simulink model "MODEL_FULL_SYSTEM"  (Simulink 7.8)
settings: Solver=ode1  StartTime=0.0  StopTime=inf  FixedStep=Ts  MaxStep=1e-3  RelTol=1e-3
PostLoadFcn:
  | Ts=80e-6; relays_settings_init;
InitFcn:
  | Ts=80e-6; relays_settings_init;
values from neighbouring files (symbols this model uses):
  relay_sets = xlsread('relay_settings_10272015.xlsx')    [relays_settings_init.m]
undefined symbols (not defined in the file or in its folder): dfilt, DiscIntNeverNeededParam, fdesignblkfcn, gcbh, Left, opmodbus_cb, ph, Right, type, V, X
libraries: simulink x72, modbus_lib x40, cables_lib x36, rtio_opalrt_common x21, rtlab x20, transformer_lib x13, dynamic_load_lib x12, powerlib x6, simulink_extras x6, ssn_lib x5, discretizing x4, rteventslib x4
(part 6 of 7)

== system MODEL_FULL_SYSTEM/SM_Master/Generator_09222015/Woodward Inputs/Speed_System ==
  In1 : Inport
  Clock1 : Clock
      settings: DisableCoverage=on
  Duty : Constant  DisableCoverage=on  Value=0.5
  Gain1 : Gain  Gain=5
  Gain3 : Gain  Gain=5
  Gain4 : Gain  Gain=1800
  Output : Trigonometry
  Product1 : Product  DisableCoverage=on  SaturateOnIntegerOverflow=on  InputSameDT=on  OutDataTypeStr=Inherit: Same as first input
  Product3 : Product  DisableCoverage=on  SaturateOnIntegerOverflow=on  InputSameDT=on  OutDataTypeStr=Inherit: Same as first input
  RTE Conversion : rteventslib/Signal Attributes/RTE Conversion  inputdatatype=RTE Boolean  outputdatatype=Double  compensation=Disabled  nbMaxEvents=10  sampleTime=Ts
  RTE SPWM : rteventslib/Sources/RTE SPWM  NumberPhases=1-ph  CenterAlignmentMode=On  MaxFreq=inf  MinFreq=0  EnablingPort=off  ComplementaryMode=off  SpaceVector=off  RiseTimeDelay=0  MaxEvents=10  SampleTime=Ts
  initialFreq : Constant  DisableCoverage=on  Value=2*pi
  Out1 : Outport
  wires:
  Gain1/1 -> Out1/1
  RTE Conversion/1 -> Gain1/1
  Duty/1 -> RTE SPWM/2
  RTE SPWM/1 -> RTE Conversion/1
  In1/1 -> Gain4/1
  Output/1 -> Gain3/1
  Gain4/1 -> RTE SPWM/1, Product3/2
  Product3/1 -> Product1/2
  initialFreq/1 -> Product3/1
  Clock1/1 -> Product1/1
  Product1/1 -> Output/1

== system MODEL_FULL_SYSTEM/SM_Master/Generator_09222015/Woodward Inputs/Speed_System1 ==
  In1 : Inport
  Clock1 : Clock
      settings: DisableCoverage=on
  Duty : Constant  DisableCoverage=on  Value=0.5
  Gain1 : Gain  Gain=5
  Gain3 : Gain  Gain=5
  Gain4 : Gain  Gain=1800
  Output : Trigonometry
  Product1 : Product  DisableCoverage=on  SaturateOnIntegerOverflow=on  InputSameDT=on  OutDataTypeStr=Inherit: Same as first input
  Product3 : Product  DisableCoverage=on  SaturateOnIntegerOverflow=on  InputSameDT=on  OutDataTypeStr=Inherit: Same as first input
  RTE Conversion : rteventslib/Signal Attributes/RTE Conversion  inputdatatype=RTE Boolean  outputdatatype=Double  compensation=Disabled  nbMaxEvents=10  sampleTime=Ts
  RTE SPWM : rteventslib/Sources/RTE SPWM  NumberPhases=1-ph  CenterAlignmentMode=On  MaxFreq=inf  MinFreq=0  EnablingPort=off  ComplementaryMode=off  SpaceVector=off  RiseTimeDelay=0  MaxEvents=10  SampleTime=Ts
  initialFreq : Constant  DisableCoverage=on  Value=2*pi
  Out1 : Outport
  wires:
  Gain1/1 -> Out1/1
  RTE Conversion/1 -> Gain1/1
  Duty/1 -> RTE SPWM/2
  RTE SPWM/1 -> RTE Conversion/1
  In1/1 -> Gain4/1
  Output/1 -> Gain3/1
  Gain4/1 -> RTE SPWM/1, Product3/2
  Product3/1 -> Product1/2
  initialFreq/1 -> Product3/1
  Clock1/1 -> Product1/1
  Product1/1 -> Output/1

== system MODEL_FULL_SYSTEM/SM_Master/Generator_09222015/Woodward Outputs/DIO - Gr3 ==
  Dout : Inport
  Bus Creator : BusCreator  Inputs=2
  Bus Selector : BusSelector  OutputSignals=DI_CH00-07  OutputAsBus=on
  Bus Selector1 : BusSelector  OutputSignals=DI_CH08-15  OutputAsBus=on
  Conditioning : Subsystem
  Conditioning1 : Subsystem
  DigitalIn : rtio_opalrt_common/DigitalIn  CtrlName='OpCtrl'  portNb=5  FcnNos=Slot 3 Module A Subsection 1  size=1  maxcount=8  count=8  sampleTime=0  numchan=8
      settings: AttributesFormatString=%<CtrlName>
  DigitalIn1 : rtio_opalrt_common/DigitalIn  CtrlName='OpCtrl'  portNb=6  FcnNos=Slot 3 Module A Subsection 2  size=1  maxcount=8  count=8  sampleTime=0  numchan=8
      settings: AttributesFormatString=%<CtrlName>
  DigitalOut : rtio_opalrt_common/DigitalOut  CtrlName='OpCtrl'  portNb=5  FcnNos=Slot 3 Module B Subsection 1  size=1  maxcount=8  count=8  numchan=8
      settings: AttributesFormatString=%<CtrlName>
  DigitalOut1 : rtio_opalrt_common/DigitalOut  CtrlName='OpCtrl'  portNb=6  FcnNos=Slot 3 Module B Subsection 2  size=1  maxcount=8  count=8  numchan=8
      settings: AttributesFormatString=%<CtrlName>
  Terminator{1,3,5..6} (4 alike) : Terminator
  DIn : Outport
  wires:
  DigitalOut/1 -> Terminator3/1
  DigitalOut1/1 -> Terminator1/1
  Dout/1 -> Bus Selector/1, Bus Selector1/1
  Bus Selector/1 -> DigitalOut/1
  Bus Selector1/1 -> DigitalOut1/1
  DigitalIn/2 -> Terminator5/1
  DigitalIn1/2 -> Terminator6/1
  DigitalIn/1 -> Conditioning/1(In1)  "DI_CH00-07"
  DigitalIn1/1 -> Conditioning1/1(In1)  "DI_CH08-15"
  Bus Creator/1 -> DIn/1
  Conditioning/1(Out1) -> Bus Creator/1
  Conditioning1/1(Out1) -> Bus Creator/2

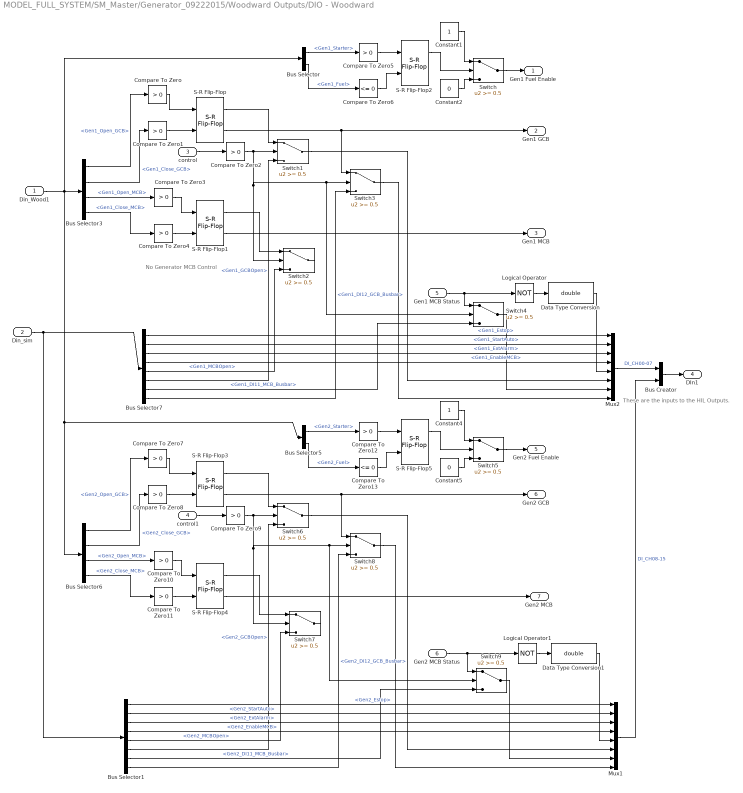
== system MODEL_FULL_SYSTEM/SM_Master/Generator_09222015/Woodward Outputs/DIO - Woodward ==
  note: No Generator MCB Control
  note: These are the inputs to
      | the HIL Outputs.
  Din_Wood1 : Inport
  Din_sim : Inport  Port=2
  control : Inport  Port=3
  control1 : Inport  Port=4
  Gen1 MCB Status : Inport  Port=5
  Gen2 MCB Status : Inport  Port=6
  Bus Creator : BusCreator  Inputs=2
  Bus Selector : BusSelector  OutputSignals=DI_CH00-07.Gen1_Starter,DI_CH00-07.Gen1_Fuel
  Bus Selector1 : BusSelector  OutputSignals=16 DOUT GR3.08-11.Gen2_Estop,16 DOUT GR3.08-11.Gen2_StartAuto,16 DOUT GR3.08-11.Gen2_ExtAlarm,16 DOUT GR3.08-11.Gen2_EnableMCB,16 DOUT GR3.12-15.Gen2_MCBOpen,16 DOUT GR3.12-15.Gen2_GCBOpen,16 DOUT GR3.12-15.Gen2_DI11_MCB_Busbar,16 DOUT GR3.12-15.Gen2_DI12_GCB_Busbar
  Bus Selector3 : BusSelector  OutputSignals=DI_CH00-07.Gen1_Open_GCB,DI_CH00-07.Gen1_Close_GCB,DI_CH00-07.Gen1_Open_MCB,DI_CH00-07.Gen1_Close_MCB
  Bus Selector5 : BusSelector  OutputSignals=DI_CH08-15.Gen2_Starter,DI_CH08-15.Gen2_Fuel
  Bus Selector6 : BusSelector  OutputSignals=DI_CH08-15.Gen2_Open_GCB,DI_CH08-15.Gen2_Close_GCB,DI_CH08-15.Gen2_Open_MCB,DI_CH08-15.Gen2_Close_MCB
  Bus Selector7 : BusSelector  OutputSignals=16 DOUT GR3.00-03.Gen1_Estop,16 DOUT GR3.00-03.Gen1_StartAuto,16 DOUT GR3.00-03.Gen1_ExtAlarm,16 DOUT GR3.00-03.Gen1_EnableMCB,16 DOUT GR3.04-07.Gen1_MCBOpen,16 DOUT GR3.04-07.Gen1_GCBOpen,16 DOUT GR3.04-07.Gen1_DI11_MCB_Busbar,16 DOUT GR3.04-07.Gen1_DI12_GCB_Busbar
  Compare To Zero{,1..5,7..12} (12 alike) : simulink/Logic and Bit Operations/Compare To Zero  relop=>  OutDataTypeStr=boolean
  Compare To Zero13 : simulink/Logic and Bit Operations/Compare To Zero  relop=<=  OutDataTypeStr=boolean
  Compare To Zero6 : simulink/Logic and Bit Operations/Compare To Zero  relop=<=  OutDataTypeStr=boolean
  Constant1 : Constant
  Constant2 : Constant  Value=0
  Constant4 : Constant
  Constant5 : Constant  Value=0
  Data Type Conversion : DataTypeConversion  OutDataTypeStr=double
  Data Type Conversion1 : DataTypeConversion  OutDataTypeStr=double
  Logical Operator : Logic  Operator=NOT  AllPortsSameDT=off  OutDataTypeStr=boolean
  Logical Operator1 : Logic  Operator=NOT  AllPortsSameDT=off  OutDataTypeStr=boolean
  Mux1 : Mux  Inputs=8
  Mux2 : Mux  Inputs=8
  S-R Flip-Flop{,1,3..4} (4 alike) : simulink_extras/Flip Flops/S-R Flip-Flop  initial_condition=1
  S-R Flip-Flop2 : simulink_extras/Flip Flops/S-R Flip-Flop  initial_condition=0
  S-R Flip-Flop5 : simulink_extras/Flip Flops/S-R Flip-Flop  initial_condition=0
  Switch : Switch  Threshold=0.5
  Switch{1..4,6..9} (8 alike) : Switch  Threshold=0.5  OutDataTypeStr=double
      Switch8 settings: LockScale=on
  Switch5 : Switch  Threshold=0.5
  Gen1 Fuel Enable : Outport
  Gen1 GCB : Outport  Port=2
  Gen1 MCB : Outport  Port=3
  DIn1 : Outport  Port=4
  Gen2 Fuel Enable : Outport  Port=5
  Gen2 GCB : Outport  Port=6
  Gen2 MCB : Outport  Port=7
  wires:
  S-R Flip-Flop1/2 -> Gen1 MCB/1
  Din_Wood1/1 -> Bus Selector3/1, Bus Selector/1, Bus Selector6/1, Bus Selector5/1
  control/1 -> Compare To Zero2/1
  Bus Creator/1 -> DIn1/1
  S-R Flip-Flop/1 -> Switch1/1
  Switch1/1 -> Mux2/6
  Bus Selector3/1 -> Compare To Zero/1  "<Gen1_Open_GCB>"
  Compare To Zero/1 -> S-R Flip-Flop/1
  Compare To Zero1/1 -> S-R Flip-Flop/2
  Bus Selector3/4 -> Compare To Zero4/1  "<Gen1_Close_MCB>"
  Compare To Zero4/1 -> S-R Flip-Flop1/2
  Compare To Zero3/1 -> S-R Flip-Flop1/1
  S-R Flip-Flop1/1 -> Switch2/1
  Compare To Zero2/1 -> Switch1/2, Switch2/2, Switch3/2, Switch4/2
  Mux1/1 -> Bus Creator/2  "DI_CH08-15"
  S-R Flip-Flop/2 -> Gen1 GCB/1, Switch3/1
  Bus Selector/1 -> Compare To Zero5/1  "<Gen1_Starter>"
  Bus Selector/2 -> Compare To Zero6/1  "<Gen1_Fuel>"
  S-R Flip-Flop2/1 -> Switch/2
  Compare To Zero5/1 -> S-R Flip-Flop2/1
  Constant2/1 -> Switch/3
  Constant1/1 -> Switch/1
  Compare To Zero6/1 -> S-R Flip-Flop2/2
  Switch/1 -> Gen1 Fuel Enable/1
  control1/1 -> Compare To Zero9/1
  S-R Flip-Flop3/1 -> Switch6/1
  Switch6/1 -> Mux1/6
  Bus Selector6/1 -> Compare To Zero7/1  "<Gen2_Open_GCB>"
  Compare To Zero7/1 -> S-R Flip-Flop3/1
  Compare To Zero8/1 -> S-R Flip-Flop3/2
  Bus Selector6/4 -> Compare To Zero11/1  "<Gen2_Close_MCB>"
  Compare To Zero11/1 -> S-R Flip-Flop4/2
  Bus Selector6/3 -> Compare To Zero10/1  "<Gen2_Open_MCB>"
  Compare To Zero10/1 -> S-R Flip-Flop4/1
  S-R Flip-Flop4/1 -> Switch7/1
  Bus Selector6/2 -> Compare To Zero8/1  "<Gen2_Close_GCB>"
  Compare To Zero9/1 -> Switch6/2, Switch7/2, Switch8/2, Switch9/2
  S-R Flip-Flop3/2 -> Gen2 GCB/1, Switch8/1
  S-R Flip-Flop4/2 -> Gen2 MCB/1
  Bus Selector5/1 -> Compare To Zero12/1  "<Gen2_Starter>"
  Bus Selector5/2 -> Compare To Zero13/1  "<Gen2_Fuel>"
  S-R Flip-Flop5/1 -> Switch5/2
  Compare To Zero12/1 -> S-R Flip-Flop5/1
  Constant5/1 -> Switch5/3
  Constant4/1 -> Switch5/1
  Compare To Zero13/1 -> S-R Flip-Flop5/2
  Switch5/1 -> Gen2 Fuel Enable/1
  Bus Selector3/2 -> Compare To Zero1/1  "<Gen1_Close_GCB>"
  Bus Selector3/3 -> Compare To Zero3/1  "<Gen1_Open_MCB>"
  Bus Selector1/1 -> Mux1/1  "<Gen2_Estop>"
  Bus Selector1/2 -> Mux1/2  "<Gen2_StartAuto>"
  Bus Selector1/3 -> Mux1/3  "<Gen2_ExtAlarm>"
  Bus Selector1/4 -> Mux1/4  "<Gen2_EnableMCB>"
  Bus Selector1/5 -> Switch7/3  "<Gen2_MCBOpen>"
  Bus Selector1/6 -> Switch6/3  "<Gen2_GCBOpen>"
  Bus Selector7/1 -> Mux2/1  "<Gen1_Estop>"
  Bus Selector7/2 -> Mux2/2  "<Gen1_StartAuto>"
  Bus Selector7/3 -> Mux2/3  "<Gen1_ExtAlarm>"
  Bus Selector7/4 -> Mux2/4  "<Gen1_EnableMCB>"
  Bus Selector7/5 -> Switch2/3  "<Gen1_MCBOpen>"
  Bus Selector7/6 -> Switch1/3  "<Gen1_GCBOpen>"
  Mux2/1 -> Bus Creator/1  "DI_CH00-07"
  Din_sim/1 -> Bus Selector7/1, Bus Selector1/1
  Bus Selector7/7 -> Switch4/3  "<Gen1_DI11_MCB_Busbar>"
  Switch4/1 -> Mux2/7
  Bus Selector7/8 -> Switch3/3  "<Gen1_DI12_GCB_Busbar>"
  Switch3/1 -> Mux2/8
  Bus Selector1/7 -> Switch9/3  "<Gen2_DI11_MCB_Busbar>"
  Switch9/1 -> Mux1/7
  Bus Selector1/8 -> Switch8/3  "<Gen2_DI12_GCB_Busbar>"
  Switch8/1 -> Mux1/8
  Gen1 MCB Status/1 -> Logical Operator/1, Switch4/1
  Data Type Conversion/1 -> Mux2/5
  Logical Operator/1 -> Data Type Conversion/1
  Gen2 MCB Status/1 -> Logical Operator1/1, Switch9/1
  Logical Operator1/1 -> Data Type Conversion1/1
  Data Type Conversion1/1 -> Mux1/5

== system MODEL_FULL_SYSTEM/SM_Master/Generator_09222015/Woodward Outputs/DOUT type config ==
  note: The Constants are used to select Digital Output type:
      | - 0: Time-Stamped Digital Output
      | - 1: Pulse-Width Modulated DIgital Output
  DataIn Send : rtio_opalrt_common/DataIn Send  CtrlName='OpCtrl'  FcnNos=11  width=1  portType=double  checkVersion=off  expectedId=0  expectedVersion=0  opComp=>=
      settings: AttributesFormatString=%<CtrlName>
  DataIn Send1 : rtio_opalrt_common/DataIn Send  CtrlName='OpCtrl'  FcnNos=12  width=1  portType=double  checkVersion=off  expectedId=0  expectedVersion=0  opComp=>=
      settings: AttributesFormatString=%<CtrlName>
  Subsection 3 DOUT type : Constant
  Subsection 4 DOUT type : Constant
  Terminator1 : Terminator
  Terminator2 : Terminator
  wires:
  Subsection 3 DOUT type/1 -> DataIn Send/1
  Subsection 4 DOUT type/1 -> DataIn Send1/1
  DataIn Send1/1 -> Terminator1/1
  DataIn Send/1 -> Terminator2/1

== system MODEL_FULL_SYSTEM/SM_Master/Generator_09222015/Woodward Outputs/PWM IO - Gr3 ==
  PWMOut : Inport
  Bus Creator : BusCreator  Inputs=2
  Bus Creator1 : BusCreator  Inputs=2
  Bus Creator2 : BusCreator  Inputs=2
  Bus Selector : BusSelector  OutputSignals=FreqPWMOut16-23,DutyPWMOut16-23
  Bus Selector1 : BusSelector  OutputSignals=FreqPWMOut24-31,DutyPWMOut24-31
  Bus Selector2 : BusSelector  OutputSignals=16 PWMOUT GR3.Ch16-23,16 PWMOUT GR3.Ch24-31
  PWM In : rtio_opalrt_common/PWM In  CtrlName='OpCtrl'  portNb=9  FcnNos=Slot 3 Module A Subsection 3  maxCount=8  Count=8  sampleTime=0  numchan=8
      settings: AttributesFormatString=%<CtrlName>
  PWM In1 : rtio_opalrt_common/PWM In  CtrlName='OpCtrl'  portNb=10  FcnNos=Slot 3 Module A Subsection 4  maxCount=8  Count=8  sampleTime=0  numchan=8
      settings: AttributesFormatString=%<CtrlName>
  PWM Out : rtio_opalrt_common/PWM Out  CtrlName='OpCtrl'  portNb=9  FcnNos=Slot 3 Module B Subsection 3  size=64  maxcount=8  count=8  polarity=Active High  symMode=Symmetric  complementary=off  deadTime=0  numchan=8  loadnb=1  initphase=[0 0 0 0 0 0 0 0]
      settings: AttributesFormatString=%<CtrlName>
  PWM Out1 : rtio_opalrt_common/PWM Out  CtrlName='OpCtrl'  portNb=10  FcnNos=Slot 3 Module B Subsection 4  size=64  maxcount=8  count=8  polarity=Active High  symMode=Symmetric  complementary=off  deadTime=0  numchan=8  loadnb=2  initphase=[0 0 0 0 0 0 0 0]
      settings: AttributesFormatString=%<CtrlName>
  Terminator{,1,4..5} (4 alike) : Terminator
  PWMIn : Outport
  wires:
  Bus Selector/1 -> PWM Out/1  "<FreqPWMOut16-23>"
  Bus Selector/2 -> PWM Out/2  "<DutyPWMOut16-23>"
  PWM Out/1 -> Terminator/1
  Bus Selector1/1 -> PWM Out1/1  "<FreqPWMOut24-31>"
  Bus Selector1/2 -> PWM Out1/2  "<DutyPWMOut24-31>"
  PWM Out1/1 -> Terminator1/1
  PWMOut/1 -> Bus Selector2/1
  Bus Selector2/1 -> Bus Selector/1  "<Ch16-23>"
  Bus Creator/1 -> PWMIn/1
  Bus Creator1/1 -> Bus Creator/1  "PWMI_CH16-23"
  Bus Creator2/1 -> Bus Creator/2  "PWMI_CH24-31"
  PWM In1/3 -> Terminator5/1
  PWM In/3 -> Terminator4/1
  PWM In/1 -> Bus Creator1/1  "Freq"
  PWM In/2 -> Bus Creator1/2  "Duty"
  PWM In1/1 -> Bus Creator2/1  "Freq"
  PWM In1/2 -> Bus Creator2/2  "Duty"
  Bus Selector2/2 -> Bus Selector1/1  "<Ch24-31>"

== system MODEL_FULL_SYSTEM/SM_Master/Generator_09222015/Woodward Outputs/TSDIO - Gr3 ==
  TSDout : Inport
  Bus Creator : BusCreator  Inputs=16
  Bus Creator1 : BusCreator  Inputs=16
  Bus Creator2 : BusCreator  Inputs=2
  Bus Selector : BusSelector  OutputSignals=16 TSDOUT GR3.states.CH16-23.states 17,16 TSDOUT GR3.times CH16-23.times17,16 TSDOUT GR3.states.CH16-23.states 18,16 TSDOUT GR3.times CH16-23.times18,16 TSDOUT GR3.states.CH16-23.states 19,16 TSDOUT GR3.times CH16-23.times19,16 TSDOUT GR3.states.CH16-23.states 20,16 TSDOUT GR3.times CH16-23.times20,16 TSDOUT GR3.states.CH16-23.states 21,16 TSDOUT GR3.times CH16-23.times21,16 TSDOUT GR3.states.CH16-23.states 22,16 TSDOUT GR3.times CH16-23.times22,16 TSDOUT GR3.states.CH16-23.states 23,16 TSDOUT GR3.times CH16-23.times23,16 TSDOUT GR3.states.CH16-23.states 24,16 TSDOUT GR3.times CH16-23.times24
  Bus Selector1 : BusSelector  OutputSignals=16 TSDOUT GR3.states.CH24-31.states 25,16 TSDOUT GR3.times CH24-31.times25,16 TSDOUT GR3.states.CH24-31.states 26,16 TSDOUT GR3.times CH24-31.times26,16 TSDOUT GR3.states.CH24-31.states 27,16 TSDOUT GR3.times CH24-31.times27,16 TSDOUT GR3.states.CH24-31.states 28,16 TSDOUT GR3.times CH24-31.times28,16 TSDOUT GR3.states.CH24-31.states 29,16 TSDOUT GR3.times CH24-31.times29,16 TSDOUT GR3.states.CH24-31.states 30,16 TSDOUT GR3.times CH24-31.times30,16 TSDOUT GR3.states.CH24-31.states 31,16 TSDOUT GR3.times CH24-31.times31,16 TSDOUT GR3.states.CH24-31.states 32,16 TSDOUT GR3.times CH24-31.times32
  EventDetector : rtio_opalrt_common/EventDetector  CtrlName='OpCtrl'  portNb=7  FcnNos=Slot 3 Module A Subsection 3  size=32  maxcount=8  nbChannels=8  width=4  timeUnit=Time ratio  sampleTime=0  numwidth=4
      settings: AttributesFormatString=%<CtrlName>
  EventDetector1 : rtio_opalrt_common/EventDetector  CtrlName='OpCtrl'  portNb=8  FcnNos=Slot 3 Module A Subsection 4  size=32  maxcount=8  nbChannels=8  width=4  timeUnit=Time ratio  sampleTime=0  numwidth=4
      settings: AttributesFormatString=%<CtrlName>
  EventGenerator : rtio_opalrt_common/EventGenerator  CtrlName='OpCtrl'  portNb=7  FcnNos=Slot 3 Module B Subsection 3  size=32  count=8  nbChannels=8  width=4  timeUnit=Time ratio  numwidth=4
      settings: AttributesFormatString=%<CtrlName>
  EventGenerator1 : rtio_opalrt_common/EventGenerator  CtrlName='OpCtrl'  portNb=8  FcnNos=Slot 3 Module B Subsection 4  size=32  count=8  nbChannels=8  width=4  timeUnit=Time ratio  numwidth=4
      settings: AttributesFormatString=%<CtrlName>
  Terminator{,1..3} (4 alike) : Terminator
  TSDin : Outport
  wires:
  TSDout/1 -> Bus Selector/1, Bus Selector1/1
  Bus Selector/16 -> EventGenerator/16  "<times24>"
  Bus Selector/15 -> EventGenerator/15  "<states 24>"
  Bus Selector/14 -> EventGenerator/14  "<times23>"
  Bus Selector/13 -> EventGenerator/13  "<states 23>"
  Bus Selector/12 -> EventGenerator/12  "<times22>"
  Bus Selector/11 -> EventGenerator/11  "<states 22>"
  Bus Selector/10 -> EventGenerator/10  "<times21>"
  Bus Selector/9 -> EventGenerator/9  "<states 21>"
  Bus Selector/8 -> EventGenerator/8  "<times20>"
  Bus Selector/7 -> EventGenerator/7  "<states 20>"
  Bus Selector/6 -> EventGenerator/6  "<times19>"
  Bus Selector/5 -> EventGenerator/5  "<states 19>"
  Bus Selector/4 -> EventGenerator/4  "<times18>"
  Bus Selector/3 -> EventGenerator/3  "<states 18>"
  Bus Selector/2 -> EventGenerator/2  "<times17>"
  Bus Selector/1 -> EventGenerator/1  "<states 17>"
  EventGenerator/1 -> Terminator/1
  EventDetector/16 -> Bus Creator/16  "times8"
  EventDetector/15 -> Bus Creator/15  "states8"
  EventDetector/14 -> Bus Creator/14  "times7"
  EventDetector/13 -> Bus Creator/13  "states7"
  EventDetector/12 -> Bus Creator/12  "times6"
  EventDetector/11 -> Bus Creator/11  "states6"
  EventDetector/10 -> Bus Creator/10  "times5"
  EventDetector/9 -> Bus Creator/9  "states5"
  EventDetector/8 -> Bus Creator/8  "times4"
  EventDetector/7 -> Bus Creator/7  "states4"
  EventDetector/6 -> Bus Creator/6  "times3"
  EventDetector/5 -> Bus Creator/5  "states3"
  EventDetector/4 -> Bus Creator/4  "times2"
  EventDetector/3 -> Bus Creator/3  "states2"
  EventDetector/2 -> Bus Creator/2  "times1"
  EventDetector/1 -> Bus Creator/1  "states1"
  EventDetector/17 -> Terminator1/1
  EventGenerator1/1 -> Terminator2/1
  Bus Selector1/1 -> EventGenerator1/1  "<states 25>"
  Bus Selector1/2 -> EventGenerator1/2  "<times25>"
  Bus Selector1/3 -> EventGenerator1/3  "<states 26>"
  Bus Selector1/4 -> EventGenerator1/4  "<times26>"
  Bus Selector1/5 -> EventGenerator1/5  "<states 27>"
  Bus Selector1/6 -> EventGenerator1/6  "<times27>"
  Bus Selector1/7 -> EventGenerator1/7  "<states 28>"
  Bus Selector1/8 -> EventGenerator1/8  "<times28>"
  Bus Selector1/9 -> EventGenerator1/9  "<states 29>"
  Bus Selector1/10 -> EventGenerator1/10  "<times29>"
  Bus Selector1/11 -> EventGenerator1/11  "<states 30>"
  Bus Selector1/12 -> EventGenerator1/12  "<times30>"
  Bus Selector1/13 -> EventGenerator1/13  "<states 31>"
  Bus Selector1/14 -> EventGenerator1/14  "<times31>"
  Bus Selector1/15 -> EventGenerator1/15  "<states 32>"
  Bus Selector1/16 -> EventGenerator1/16  "<times32>"
  Bus Creator1/1 -> Bus Creator2/2  "CH24-31"
  EventDetector1/16 -> Bus Creator1/16  "times6"
  EventDetector1/15 -> Bus Creator1/15  "states6"
  EventDetector1/14 -> Bus Creator1/14  "times5"
  EventDetector1/13 -> Bus Creator1/13  "states5"
  EventDetector1/12 -> Bus Creator1/12  "times4"
  EventDetector1/11 -> Bus Creator1/11  "states4"
  EventDetector1/10 -> Bus Creator1/10  "times3"
  EventDetector1/9 -> Bus Creator1/9  "states3"
  EventDetector1/8 -> Bus Creator1/8  "times2"
  EventDetector1/7 -> Bus Creator1/7  "states2"
  EventDetector1/6 -> Bus Creator1/6  "times1"
  EventDetector1/5 -> Bus Creator1/5  "states1"
  EventDetector1/4 -> Bus Creator1/4  "times2"
  EventDetector1/3 -> Bus Creator1/3  "states2"
  EventDetector1/2 -> Bus Creator1/2  "times1"
  EventDetector1/1 -> Bus Creator1/1  "states1"
  EventDetector1/17 -> Terminator3/1  "states7"
  Bus Creator/1 -> Bus Creator2/1  "CH16-23"
  Bus Creator2/1 -> TSDin/1  "TSDIN"

== system MODEL_FULL_SYSTEM/SM_Master/Generator_09222015/Woodward Outputs/Woodward Primary Inputs ==
  Bias-ctrl : Inport
  Bus Creator : BusCreator
  Bus Creator1 : BusCreator
  Constant{,5,10..11} (4 alike) : Constant  Value=1.00
  Constant{1,3..4,6,8..9} (6 alike) : Constant  Value=0
  Constant2 : Constant  Value=20
  Constant7 : Constant  Value=20
  Demux1 : Demux  Outputs=16
  Divide{,1..3} (4 alike) : Product  Inputs=*/
  GR1 B AIN (CH00-15) : Subsystem
  Lowpass Filter : Subsystem  DialogController=fdesignblkfcn  DialogControllerArgs=DataTag4  InitFcn=fdesignblkfcn(gcbh, {'InitFcn'});
      settings: CopyFcn=fdesignblkfcn(gcbh, {'CopyFcn'});
      mask Type: Lowpass Filter
      mask Description: Design a lowpass filter
      mask Help: helpview(mapfilelocation('dsp'), 'dsplowpassfilter');
      mask Display: disp('Lowpass')
  Lowpass Filter1 : Subsystem  DialogController=fdesignblkfcn  DialogControllerArgs=DataTag7  InitFcn=fdesignblkfcn(gcbh, {'InitFcn'});
      settings: CopyFcn=fdesignblkfcn(gcbh, {'CopyFcn'});
      mask Type: Lowpass Filter
      mask Description: Design a lowpass filter
      mask Help: helpview(mapfilelocation('dsp'), 'dsplowpassfilter');
      mask Display: disp('Lowpass')
  Lowpass Filter2 : Subsystem  DialogController=fdesignblkfcn  DialogControllerArgs=DataTag10  InitFcn=fdesignblkfcn(gcbh, {'InitFcn'});
      settings: CopyFcn=fdesignblkfcn(gcbh, {'CopyFcn'});
      mask Type: Lowpass Filter
      mask Description: Design a lowpass filter
      mask Help: helpview(mapfilelocation('dsp'), 'dsplowpassfilter');
      mask Display: disp('Lowpass')
  Lowpass Filter3 : Subsystem  DialogController=fdesignblkfcn  DialogControllerArgs=DataTag13  InitFcn=fdesignblkfcn(gcbh, {'InitFcn'});
      settings: CopyFcn=fdesignblkfcn(gcbh, {'CopyFcn'});
      mask Type: Lowpass Filter
      mask Description: Design a lowpass filter
      mask Help: helpview(mapfilelocation('dsp'), 'dsplowpassfilter');
      mask Display: disp('Lowpass')
  Sum{,1..3} (4 alike) : Sum  Inputs=|+-
  Switch{,1..3} (4 alike) : Switch  Threshold=0.5
  Gen1 Gov and AVR : Outport
  Gen2 Gov and AVR : Outport  Port=2
  wires:
  GR1 B AIN (CH00-15)/1(Out1) -> [AINs_Gr1], Demux1/1
  Demux1/1 -> Divide/1
  Demux1/2 -> Divide1/1
  Constant2/1 -> Divide1/2, Divide/2
  Divide/1 -> Sum/1
  Divide1/1 -> Sum1/1
  Constant3/1 -> Sum/2
  Constant4/1 -> Sum1/2
  Sum/1 -> Lowpass Filter/1(In)
  Switch/1 -> Bus Creator/3  "Gen1 Gov"
  Switch1/1 -> Bus Creator/4  "Gen1 AVR"
  Sum1/1 -> Lowpass Filter1/1(In)
  Constant1/1 -> Switch/3, Switch1/3
  Bias-ctrl/1 -> Switch/2, Switch1/2, Switch2/2, Switch3/2
  Lowpass Filter/1(Out) -> Switch/1
  Lowpass Filter1/1(Out) -> Switch1/1
  Constant5/1 -> Bus Creator/2  "Gen1 Ref AVR"
  Constant/1 -> Bus Creator/1  "Gen1 Ref GOV"
  Demux1/3 -> Divide2/1
  Demux1/4 -> Divide3/1
  Constant7/1 -> Divide3/2, Divide2/2
  Divide2/1 -> Sum2/1
  Divide3/1 -> Sum3/1
  Constant8/1 -> Sum2/2
  Constant9/1 -> Sum3/2
  Sum2/1 -> Lowpass Filter2/1(In)
  Switch2/1 -> Bus Creator1/3  "Gen2 GOV"
  Switch3/1 -> Bus Creator1/4  "Gen2 AVR"
  Sum3/1 -> Lowpass Filter3/1(In)
  Constant6/1 -> Switch2/3, Switch3/3
  Lowpass Filter2/1(Out) -> Switch2/1
  Lowpass Filter3/1(Out) -> Switch3/1
  Constant11/1 -> Bus Creator1/2  "Gen2 Ref AVR"
  Constant10/1 -> Bus Creator1/1  "Gen2 Ref GOV"
  Bus Creator/1 -> Gen1 Gov and AVR/1
  Bus Creator1/1 -> Gen2 Gov and AVR/1

== system MODEL_FULL_SYSTEM/SC_Console/Woodward2/16TSDIn/16 TSDOut GR3/Dout state ctrl/Dout_CH16_CH23 ==
  Bus Creator1 : BusCreator  Inputs=8
  Dout_CH{16..23} (8 alike) : Constant  Value=[1 0 1 0]
  Manual Switch{17..24} (8 alike) : simulink/Signal Routing/Manual Switch  sw=1  action=0  varsize=off
  Zero_Dout_CH{16..23} (8 alike) : Constant  Value=[0 0 0 0]
  Dout_CH8_CH15 : Outport
  wires:
  Manual Switch24/1 -> Bus Creator1/8  "states 24"
  Manual Switch23/1 -> Bus Creator1/7  "states 23"
  Manual Switch22/1 -> Bus Creator1/6  "states 22"
  Manual Switch21/1 -> Bus Creator1/5  "states 21"
  Manual Switch20/1 -> Bus Creator1/4  "states 20"
  Manual Switch19/1 -> Bus Creator1/3  "states 19"
  Manual Switch18/1 -> Bus Creator1/2  "states 18"
  Manual Switch17/1 -> Bus Creator1/1  "states 17"
  Zero_Dout_CH23/1 -> Manual Switch24/2
  Dout_CH23/1 -> Manual Switch24/1
  Zero_Dout_CH22/1 -> Manual Switch23/2
  Dout_CH22/1 -> Manual Switch23/1
  Zero_Dout_CH21/1 -> Manual Switch22/2
  Dout_CH21/1 -> Manual Switch22/1
  Zero_Dout_CH20/1 -> Manual Switch21/2
  Dout_CH20/1 -> Manual Switch21/1
  Zero_Dout_CH19/1 -> Manual Switch20/2
  Dout_CH19/1 -> Manual Switch20/1
  Zero_Dout_CH18/1 -> Manual Switch19/2
  Dout_CH18/1 -> Manual Switch19/1
  Zero_Dout_CH17/1 -> Manual Switch18/2
  Dout_CH17/1 -> Manual Switch18/1
  Zero_Dout_CH16/1 -> Manual Switch17/2
  Dout_CH16/1 -> Manual Switch17/1
  Bus Creator1/1 -> Dout_CH8_CH15/1

== system MODEL_FULL_SYSTEM/SC_Console/Woodward2/16TSDIn/16 TSDOut GR3/Dout state ctrl/Dout_CH24_CH31 ==
  Bus Creator : BusCreator  Inputs=8
  Dout_CH{24..31} (8 alike) : Constant  Value=[1 0 1 0]
  Manual Switch{25..32} (8 alike) : simulink/Signal Routing/Manual Switch  sw=1  action=0  varsize=off
  Zero_Dout_CH{24..31} (8 alike) : Constant  Value=[0 0 0 0]
  Dout_CH8_CH15 : Outport
  wires:
  Bus Creator/1 -> Dout_CH8_CH15/1
  Dout_CH24/1 -> Manual Switch25/1
  Zero_Dout_CH24/1 -> Manual Switch25/2
  Dout_CH25/1 -> Manual Switch26/1
  Zero_Dout_CH25/1 -> Manual Switch26/2
  Dout_CH26/1 -> Manual Switch27/1
  Zero_Dout_CH26/1 -> Manual Switch27/2
  Dout_CH27/1 -> Manual Switch28/1
  Zero_Dout_CH27/1 -> Manual Switch28/2
  Dout_CH28/1 -> Manual Switch29/1
  Zero_Dout_CH28/1 -> Manual Switch29/2
  Dout_CH29/1 -> Manual Switch30/1
  Zero_Dout_CH29/1 -> Manual Switch30/2
  Dout_CH30/1 -> Manual Switch31/1
  Zero_Dout_CH30/1 -> Manual Switch31/2
  Dout_CH31/1 -> Manual Switch32/1
  Zero_Dout_CH31/1 -> Manual Switch32/2
  Manual Switch25/1 -> Bus Creator/1  "states 25"
  Manual Switch26/1 -> Bus Creator/2  "states 26"
  Manual Switch27/1 -> Bus Creator/3  "states 27"
  Manual Switch28/1 -> Bus Creator/4  "states 28"
  Manual Switch29/1 -> Bus Creator/5  "states 29"
  Manual Switch30/1 -> Bus Creator/6  "states 30"
  Manual Switch31/1 -> Bus Creator/7  "states 31"
  Manual Switch32/1 -> Bus Creator/8  "states 32"

== system MODEL_FULL_SYSTEM/SM_Master/Generator_09222015/GenSet_1MVA_09082015/900kW Generator with  Primary Controllers/Diesel Engine Speed & Voltage Control fast ==
  note: This is the device analog output of =-10Vdc to
      | the HIL Analog Input it should be scaled to 1 pu
  note: These biases may need to
      | go to the references as opposed
      | to the measured signal.
  note: originally ++
  note: originally ++
  wref : Inport  SampleTime=Ts
  Vtref : Inport  Port=2  SampleTime=Ts
  Generator Enable : Inport  Port=3  SampleTime=Ts
  m : Inport  Port=4  SampleTime=Ts
  w_meas_Wood : Inport  Port=5  SampleTime=Ts
  V_meas_Wood : Inport  Port=6  SampleTime=Ts
  Woodward Enable : Inport  Port=7  SampleTime=Ts
  Bus Creator : BusCreator  Inputs=2
  Bus Creator1 : BusCreator  Inputs=2
  Bus Creator2 : BusCreator  Inputs=2
  Bus Selector : BusSelector  OutputSignals="Mechanical.Rotor speed  wm (pu)"
  Bus Selector1 : BusSelector  OutputSignals="dq0 components.Stator voltage  vd (pu),dq0 components.Stator voltage  vq (pu)"  OutputAsBus=on
  Bus to Vector : BusToVector
  Constant1 : Constant  Value=0
  Constant2 : Constant  Value=0
  Discrete PID Controller1 : simulink/Continuous/PID Controller  Controller=PID  TimeDomain=Discrete-time  SampleTime=-1  IntegratorMethod=Forward Euler  FilterMethod=Forward Euler  Form=Parallel  P=1  I=0  D=0  N=100  InitialConditionSource=internal  InitialConditionForIntegrator=0  InitialConditionForFilter=0  ExternalReset=either  LimitOutput=on  UpperSaturationLimit=5  LowerSaturationLimit=-5  LinearizeAsGain=off  AntiWindupMode=none  Kb=1  TrackingMode=off  Kt=1  PParamMin=[]  PParamMax=[]  IParamMin=[]  IParamMax=[]  DParamMin=[]  DParamMax=[]  NParamMin=[]  NParamMax=[]  KbParamMin=[]  KbParamMax=[]  KtParamMin=[]  KtParamMax=[]  POutMin=[]  POutMax=[]  IOutMin=[]  IOutMax=[]  DOutMin=[]  DOutMax=[]  NOutMin=[]  NOutMax=[]  KbOutMin=[]  KbOutMax=[]  KtOutMin=[]  KtOutMax=[]  IntegratorOutMin=[]  IntegratorOutMax=[]  FilterOutMin=[]  FilterOutMax=[]  SumOutMin=[]  SumOutMax=[]  SumI1OutMin=[]  SumI1OutMax=[]  SumI2OutMin=[]  SumI2OutMax=[]  SumI3OutMin=[]  SumI3OutMax=[]  SumDOutMin=[]  SumDOutMax=[]  SaturationOutMin=[]  SaturationOutMax=[]  IntegratorContinuousStateAttributes=''  IntegratorStateMustResolveToSignalObject=off  IntegratorRTWStateStorageClass=Auto  FilterContinuousStateAttributes=''  FilterStateMustResolveToSignalObject=off  FilterRTWStateStorageClass=Auto
  Excitation : Subsystem  mask(Excitation System){tr=20e-4, reg=[ 200 2e-3 ], exc=[ 1 0.00000001 ], tgr=[ 1e-12 1e-12 ], damp=[0 1e-12 ], sat=[], lim=[ 0 5 0 ], v0=[ 0 0 ]}
      mask prompts: tr "Low-pass filter time constant Tr:"; reg "Regulator gain and time constant [ Ka  Ta ]:"; exc "Exciter  [ Ke  Te ]:"; tgr "Transient gain reduction [ Tb  Tc ]:"; damp "Damping filter gain and time constant  [ Kf  Tf  ]:"; sat "Field saturation parameters [ A B ]:"; lim "Regulator output limits and gain [ Efmin  Efmax  Kp ]:"; v0 "Initial values of terminal voltage  and field voltage [ Vt0 Vf0 ] :"
      mask help:
      | Implements an IEEE type 1 synchronous machine voltage regulator combined
      | to an exciter.
      |
      | The output of the block is the field voltage vfd, in pu,  to be applied to the Vf
      | Simulink input of a Synchronous Machine block.
      |
      | Connect the Vd and Vq measurements signals of the Synchronous Machine block
      | (signals 9 and 10)  to  the Vd and Vq inputs of the Excitation System block.
      mask Help: helpview(psbhelp);
  Fcn1 : Fcn  Expr=sqrt(u(1)^2 + u(2)^2)
  GOVERNOR & DIESEL ENGINE1 : Subsystem  mask(Diesel Engine & Governor){K=10, Ta=[0.025 0.0009 0.00574], Tlim=[0 1.1], Td=0.024, Pm0=0.0005}
      mask prompts: K "Regulator gain K:"; Ta "Actuator time constants [T4 T5 T6] (s) :"; Tlim "Torque limits [Tmin Tmax] (pu) :"; Td "Engine time delay Td (s) :"; Pm0 "Initial value of mechanical power  Pm0 (pu) :"
      mask help:
      | This block implements a diesel engine and governor system:
      | 1st and 2nd inputs: Desired and actual speed (pu)
      | Output: Diesel engine mechanical power.Motor inertia should be combined with generator.
      |
      | Actuator transfer function :
      |      Ha= (1+T4.s) / [ (s (1+T5.s)(1+T6.s) ]
      | Motor :
      |      Time delay Td
      |
      | (See reference in Tutorial Session 5)
  Ground : Ground
  Scope : Scope
      settings: YMin=-5.5  YMax=5.5
  Sum : Sum  Inputs=|++
  Sum1 : Sum  Inputs=|++
  Switch1 : Switch  Threshold=0.5
  Switch2 : Switch  Threshold=0.5
  Pm : Outport
  Vf : Outport  Port=2
  Vt : Outport  Port=3
  w : Outport  Port=4
  Misc : Outport  Port=5
  wires:
  GOVERNOR & DIESEL ENGINE1/1(Pmec (pu)) -> Pm/1  "Pmec_gov"
  Generator Enable/1 -> GOVERNOR & DIESEL ENGINE1/3(Reset), Discrete PID Controller1/2
  Bus to Vector/1 -> Fcn1/1
  Bus Selector1/1 -> Bus to Vector/1
  m/1 -> Bus Selector/1, Bus Selector1/1
  Bus Selector/1 -> Bus Creator/2, GOVERNOR & DIESEL ENGINE1/2(w (pu))  "<Rotor speed  wm (pu)>"
  V_meas_Wood/1 -> Switch2/1
  Fcn1/1 -> Bus Creator1/2, Excitation/2(v)  "vms"
  Ground/1 -> Excitation/3(vstab)
  Bus Creator/1 -> w/1
  Bus Creator1/1 -> Vt/1
  Excitation/1(Vf1) -> Discrete PID Controller1/1, Bus Creator2/1  "Vf_before"
  Discrete PID Controller1/1 -> Vf/1, Bus Creator2/2  "Vf_after"
  Bus Creator2/1 -> Scope/1, Misc/1
  Woodward Enable/1 -> Switch1/2, Switch2/2
  Switch1/1 -> Sum/1, Bus Creator/1  "wood_Gov_bias"
  w_meas_Wood/1 -> Switch1/1
  Constant2/1 -> Switch1/3
  Constant1/1 -> Switch2/3
  Switch2/1 -> Sum1/1, Bus Creator1/1  "wood_AVR_bias"
  Vtref/1 -> Sum1/2
  Sum1/1 -> Excitation/1(vref)
  wref/1 -> Sum/2
  Sum/1 -> GOVERNOR & DIESEL ENGINE1/1(wref (pu))  "wms"

== system MODEL_FULL_SYSTEM/SM_Master/Generator_09222015/GenSet_1MVA_09082015/Simulated Generator Controller 900 kW/PQ control ==
  P_ref (pu) : Inport
  P (pu) : Inport  Port=2
  Q_ref (pu) : Inport  Port=3
  Q (pu) : Inport  Port=4
  Discrete PID Controller : simulink/Continuous/PID Controller  Controller=PID  TimeDomain=Discrete-time  SampleTime=-1  IntegratorMethod=Forward Euler  FilterMethod=Forward Euler  Form=Parallel  P=0.001  I=1  D=0  N=10  InitialConditionSource=internal  InitialConditionForIntegrator=0  InitialConditionForFilter=0  ExternalReset=none  LimitOutput=on  UpperSaturationLimit=1.15  LowerSaturationLimit=0.85  LinearizeAsGain=off  AntiWindupMode=back-calculation  Kb=1  TrackingMode=off  Kt=1  PParamMin=[]  PParamMax=[]  IParamMin=[]  IParamMax=[]  DParamMin=[]  DParamMax=[]  NParamMin=[]  NParamMax=[]  KbParamMin=[]  KbParamMax=[]  KtParamMin=[]  KtParamMax=[]  POutMin=[]  POutMax=[]  IOutMin=[]  IOutMax=[]  DOutMin=[]  DOutMax=[]  NOutMin=[]  NOutMax=[]  KbOutMin=[]  KbOutMax=[]  KtOutMin=[]  KtOutMax=[]  IntegratorOutMin=[]  IntegratorOutMax=[]  FilterOutMin=[]  FilterOutMax=[]  SumOutMin=[]  SumOutMax=[]  SumI1OutMin=[]  SumI1OutMax=[]  SumI2OutMin=[]  SumI2OutMax=[]  SumI3OutMin=[]  SumI3OutMax=[]  SumDOutMin=[]  SumDOutMax=[]  SaturationOutMin=[]  SaturationOutMax=[]  IntegratorContinuousStateAttributes=''  IntegratorStateMustResolveToSignalObject=off  IntegratorRTWStateStorageClass=Auto  FilterContinuousStateAttributes=''  FilterStateMustResolveToSignalObject=off  FilterRTWStateStorageClass=Auto
  Discrete PID Controller1 : simulink/Continuous/PID Controller  Controller=PID  TimeDomain=Discrete-time  SampleTime=-1  IntegratorMethod=Forward Euler  FilterMethod=Forward Euler  Form=Parallel  P=1.2  I=2.5  D=0  N=10  InitialConditionSource=internal  InitialConditionForIntegrator=0  InitialConditionForFilter=0  ExternalReset=none  LimitOutput=on  UpperSaturationLimit=1.15  LowerSaturationLimit=0.85  LinearizeAsGain=off  AntiWindupMode=back-calculation  Kb=1  TrackingMode=off  Kt=1  PParamMin=[]  PParamMax=[]  IParamMin=[]  IParamMax=[]  DParamMin=[]  DParamMax=[]  NParamMin=[]  NParamMax=[]  KbParamMin=[]  KbParamMax=[]  KtParamMin=[]  KtParamMax=[]  POutMin=[]  POutMax=[]  IOutMin=[]  IOutMax=[]  DOutMin=[]  DOutMax=[]  NOutMin=[]  NOutMax=[]  KbOutMin=[]  KbOutMax=[]  KtOutMin=[]  KtOutMax=[]  IntegratorOutMin=[]  IntegratorOutMax=[]  FilterOutMin=[]  FilterOutMax=[]  SumOutMin=[]  SumOutMax=[]  SumI1OutMin=[]  SumI1OutMax=[]  SumI2OutMin=[]  SumI2OutMax=[]  SumI3OutMin=[]  SumI3OutMax=[]  SumDOutMin=[]  SumDOutMax=[]  SaturationOutMin=[]  SaturationOutMax=[]  IntegratorContinuousStateAttributes=''  IntegratorStateMustResolveToSignalObject=off  IntegratorRTWStateStorageClass=Auto  FilterContinuousStateAttributes=''  FilterStateMustResolveToSignalObject=off  FilterRTWStateStorageClass=Auto
  Sum : Sum  Inputs=|-+
  Sum1 : Sum  Inputs=|-+
  w_ref (pu) : Outport
  V_ref (pu) : Outport  Port=2
  wires:
  Sum/1 -> Discrete PID Controller/1
  P (pu)/1 -> Sum/1
  Discrete PID Controller/1 -> w_ref (pu)/1
  P_ref (pu)/1 -> Sum/2
  Sum1/1 -> Discrete PID Controller1/1
  Q (pu)/1 -> Sum1/1
  Discrete PID Controller1/1 -> V_ref (pu)/1
  Q_ref (pu)/1 -> Sum1/2

== system MODEL_FULL_SYSTEM/SM_Master/Generator_09222015/GenSet_1MVA_09082015/Simulated Generator Controller 900 kW/PV control ==
  P_ref (pu) : Inport
  P (pu) : Inport  Port=2
  Discrete PID Controller : simulink/Continuous/PID Controller  Controller=PID  TimeDomain=Discrete-time  SampleTime=-1  IntegratorMethod=Forward Euler  FilterMethod=Forward Euler  Form=Parallel  P=0.001  I=1  D=0  N=10  InitialConditionSource=internal  InitialConditionForIntegrator=0  InitialConditionForFilter=0  ExternalReset=none  LimitOutput=on  UpperSaturationLimit=1.15  LowerSaturationLimit=0.85  LinearizeAsGain=off  AntiWindupMode=back-calculation  Kb=1  TrackingMode=off  Kt=1  PParamMin=[]  PParamMax=[]  IParamMin=[]  IParamMax=[]  DParamMin=[]  DParamMax=[]  NParamMin=[]  NParamMax=[]  KbParamMin=[]  KbParamMax=[]  KtParamMin=[]  KtParamMax=[]  POutMin=[]  POutMax=[]  IOutMin=[]  IOutMax=[]  DOutMin=[]  DOutMax=[]  NOutMin=[]  NOutMax=[]  KbOutMin=[]  KbOutMax=[]  KtOutMin=[]  KtOutMax=[]  IntegratorOutMin=[]  IntegratorOutMax=[]  FilterOutMin=[]  FilterOutMax=[]  SumOutMin=[]  SumOutMax=[]  SumI1OutMin=[]  SumI1OutMax=[]  SumI2OutMin=[]  SumI2OutMax=[]  SumI3OutMin=[]  SumI3OutMax=[]  SumDOutMin=[]  SumDOutMax=[]  SaturationOutMin=[]  SaturationOutMax=[]  IntegratorContinuousStateAttributes=''  IntegratorStateMustResolveToSignalObject=off  IntegratorRTWStateStorageClass=Auto  FilterContinuousStateAttributes=''  FilterStateMustResolveToSignalObject=off  FilterRTWStateStorageClass=Auto
  Sum : Sum  Inputs=|-+
  w_ref (pu) : Outport
  wires:
  P_ref (pu)/1 -> Sum/2
  Discrete PID Controller/1 -> w_ref (pu)/1
  P (pu)/1 -> Sum/1
  Sum/1 -> Discrete PID Controller/1

== system MODEL_FULL_SYSTEM/SM_Master/Generator_09222015/GenSet_4MVA_09212015/4MVA Generator with  Primary Controllers1/Diesel Engine Speed & Voltage Control fast ==
  note: originally ++
  note: originally ++
  note: These biases may need to
      | go to the references as opposed
      | to the measured signal.
  note: This is the device analog output of =-10Vdc to
      | the HIL Analog Input it should be scaled to 1 pu
  wref : Inport  SampleTime=Ts
  Vtref : Inport  Port=2  SampleTime=Ts
  Generator Enable : Inport  Port=3  SampleTime=Ts
  m : Inport  Port=4  SampleTime=Ts
  w_meas_Wood : Inport  Port=5  SampleTime=Ts
  V_meas_Wood : Inport  Port=6  SampleTime=Ts
  Woodward Enable : Inport  Port=7  SampleTime=Ts
  Bus Creator : BusCreator  Inputs=2
  Bus Creator1 : BusCreator  Inputs=2
  Bus Creator2 : BusCreator  Inputs=2
  Bus Selector : BusSelector  OutputSignals="Mechanical.Rotor speed  wm (pu)"
  Bus Selector1 : BusSelector  OutputSignals="dq0 components.Stator voltage  vd (pu),dq0 components.Stator voltage  vq (pu)"  OutputAsBus=on
  Bus to Vector : BusToVector
  Constant1 : Constant  Value=0
  Constant2 : Constant  Value=0
  Discrete PID Controller1 : simulink/Continuous/PID Controller  Controller=PID  TimeDomain=Discrete-time  SampleTime=-1  IntegratorMethod=Forward Euler  FilterMethod=Forward Euler  Form=Parallel  P=1  I=0  D=0  N=100  InitialConditionSource=internal  InitialConditionForIntegrator=0  InitialConditionForFilter=0  ExternalReset=either  LimitOutput=on  UpperSaturationLimit=5  LowerSaturationLimit=-5  LinearizeAsGain=off  AntiWindupMode=none  Kb=1  TrackingMode=off  Kt=1  PParamMin=[]  PParamMax=[]  IParamMin=[]  IParamMax=[]  DParamMin=[]  DParamMax=[]  NParamMin=[]  NParamMax=[]  KbParamMin=[]  KbParamMax=[]  KtParamMin=[]  KtParamMax=[]  POutMin=[]  POutMax=[]  IOutMin=[]  IOutMax=[]  DOutMin=[]  DOutMax=[]  NOutMin=[]  NOutMax=[]  KbOutMin=[]  KbOutMax=[]  KtOutMin=[]  KtOutMax=[]  IntegratorOutMin=[]  IntegratorOutMax=[]  FilterOutMin=[]  FilterOutMax=[]  SumOutMin=[]  SumOutMax=[]  SumI1OutMin=[]  SumI1OutMax=[]  SumI2OutMin=[]  SumI2OutMax=[]  SumI3OutMin=[]  SumI3OutMax=[]  SumDOutMin=[]  SumDOutMax=[]  SaturationOutMin=[]  SaturationOutMax=[]  IntegratorContinuousStateAttributes=''  IntegratorStateMustResolveToSignalObject=off  IntegratorRTWStateStorageClass=Auto  FilterContinuousStateAttributes=''  FilterStateMustResolveToSignalObject=off  FilterRTWStateStorageClass=Auto
  Excitation : Subsystem  mask(Excitation System){tr=20e-4, reg=[ 200 2e-3 ], exc=[ 1 0.00000001 ], tgr=[ 1e-12 1e-12 ], damp=[0 1e-12 ], sat=[], lim=[ 0 5 0 ], v0=[ 0 0 ]}
      mask prompts: tr "Low-pass filter time constant Tr:"; reg "Regulator gain and time constant [ Ka  Ta ]:"; exc "Exciter  [ Ke  Te ]:"; tgr "Transient gain reduction [ Tb  Tc ]:"; damp "Damping filter gain and time constant  [ Kf  Tf  ]:"; sat "Field saturation parameters [ A B ]:"; lim "Regulator output limits and gain [ Efmin  Efmax  Kp ]:"; v0 "Initial values of terminal voltage  and field voltage [ Vt0 Vf0 ] :"
      mask help:
      | Implements an IEEE type 1 synchronous machine voltage regulator combined
      | to an exciter.
      |
      | The output of the block is the field voltage vfd, in pu,  to be applied to the Vf
      | Simulink input of a Synchronous Machine block.
      |
      | Connect the Vd and Vq measurements signals of the Synchronous Machine block
      | (signals 9 and 10)  to  the Vd and Vq inputs of the Excitation System block.
      mask Help: helpview(psbhelp);
  Fcn1 : Fcn  Expr=sqrt(u(1)^2 + u(2)^2)
  GOVERNOR & DIESEL ENGINE1 : Subsystem  mask(Diesel Engine & Governor){K=10, Ta=[0.025 0.0009 0.00574], Tlim=[0 1.1], Td=0.024, Pm0=0.00005}
      mask prompts: K "Regulator gain K:"; Ta "Actuator time constants [T4 T5 T6] (s) :"; Tlim "Torque limits [Tmin Tmax] (pu) :"; Td "Engine time delay Td (s) :"; Pm0 "Initial value of mechanical power  Pm0 (pu) :"
      mask help:
      | This block implements a diesel engine and governor system:
      | 1st and 2nd inputs: Desired and actual speed (pu)
      | Output: Diesel engine mechanical power.Motor inertia should be combined with generator.
      |
      | Actuator transfer function :
      |      Ha= (1+T4.s) / [ (s (1+T5.s)(1+T6.s) ]
      | Motor :
      |      Time delay Td
      |
      | (See reference in Tutorial Session 5)
  Ground : Ground
  Sum : Sum  Inputs=|++
  Sum1 : Sum  Inputs=|++
  Switch1 : Switch  Threshold=0.5
  Switch2 : Switch  Threshold=0.5
  Pm : Outport
  Vf : Outport  Port=2
  Vt : Outport  Port=3
  w : Outport  Port=4
  Misc : Outport  Port=5
  wires:
  Sum/1 -> GOVERNOR & DIESEL ENGINE1/1(wref (pu))  "wms"
  wref/1 -> Sum/2
  Sum1/1 -> Excitation/1(vref)
  Vtref/1 -> Sum1/2
  Switch2/1 -> Bus Creator1/1, Sum1/1  "wood_AVR_bias"
  Constant1/1 -> Switch2/3
  Constant2/1 -> Switch1/3
  w_meas_Wood/1 -> Switch1/1
  Switch1/1 -> Bus Creator/1, Sum/1  "wood_Gov_bias"
  Woodward Enable/1 -> Switch2/2, Switch1/2
  Bus Creator2/1 -> Misc/1
  Discrete PID Controller1/1 -> Bus Creator2/2, Vf/1  "Vf_after"
  Excitation/1(Vf1) -> Bus Creator2/1, Discrete PID Controller1/1  "Vf_before"
  Bus Creator1/1 -> Vt/1
  Bus Creator/1 -> w/1
  Ground/1 -> Excitation/3(vstab)
  Fcn1/1 -> Excitation/2(v), Bus Creator1/2  "vms"
  V_meas_Wood/1 -> Switch2/1
  Bus Selector/1 -> GOVERNOR & DIESEL ENGINE1/2(w (pu)), Bus Creator/2  "<Rotor speed  wm (pu)>"
  m/1 -> Bus Selector1/1, Bus Selector/1
  Bus Selector1/1 -> Bus to Vector/1
  Bus to Vector/1 -> Fcn1/1
  Generator Enable/1 -> Discrete PID Controller1/2, GOVERNOR & DIESEL ENGINE1/3(Reset)
  GOVERNOR & DIESEL ENGINE1/1(Pmec (pu)) -> Pm/1  "Pmec_gov"

== system MODEL_FULL_SYSTEM/SM_Master/Generator_09222015/GenSet_4MVA_09212015/Simulated Generator Controller 3.5 MW/PQ control ==
  P_ref (pu) : Inport
  P (pu) : Inport  Port=2
  Q_ref (pu) : Inport  Port=3
  Q (pu) : Inport  Port=4
  Discrete PID Controller : simulink/Continuous/PID Controller  Controller=PID  TimeDomain=Discrete-time  SampleTime=-1  IntegratorMethod=Forward Euler  FilterMethod=Forward Euler  Form=Parallel  P=0.025  I=1  D=0  N=10  InitialConditionSource=internal  InitialConditionForIntegrator=0  InitialConditionForFilter=0  ExternalReset=none  LimitOutput=on  UpperSaturationLimit=1.15  LowerSaturationLimit=0.85  LinearizeAsGain=off  AntiWindupMode=back-calculation  Kb=1  TrackingMode=off  Kt=1  PParamMin=[]  PParamMax=[]  IParamMin=[]  IParamMax=[]  DParamMin=[]  DParamMax=[]  NParamMin=[]  NParamMax=[]  KbParamMin=[]  KbParamMax=[]  KtParamMin=[]  KtParamMax=[]  POutMin=[]  POutMax=[]  IOutMin=[]  IOutMax=[]  DOutMin=[]  DOutMax=[]  NOutMin=[]  NOutMax=[]  KbOutMin=[]  KbOutMax=[]  KtOutMin=[]  KtOutMax=[]  IntegratorOutMin=[]  IntegratorOutMax=[]  FilterOutMin=[]  FilterOutMax=[]  SumOutMin=[]  SumOutMax=[]  SumI1OutMin=[]  SumI1OutMax=[]  SumI2OutMin=[]  SumI2OutMax=[]  SumI3OutMin=[]  SumI3OutMax=[]  SumDOutMin=[]  SumDOutMax=[]  SaturationOutMin=[]  SaturationOutMax=[]  IntegratorContinuousStateAttributes=''  IntegratorStateMustResolveToSignalObject=off  IntegratorRTWStateStorageClass=Auto  FilterContinuousStateAttributes=''  FilterStateMustResolveToSignalObject=off  FilterRTWStateStorageClass=Auto
  Discrete PID Controller1 : simulink/Continuous/PID Controller  Controller=PID  TimeDomain=Discrete-time  SampleTime=-1  IntegratorMethod=Forward Euler  FilterMethod=Forward Euler  Form=Parallel  P=0.2  I=1.5  D=0  N=10  InitialConditionSource=internal  InitialConditionForIntegrator=0  InitialConditionForFilter=0  ExternalReset=none  LimitOutput=on  UpperSaturationLimit=1.15  LowerSaturationLimit=0.85  LinearizeAsGain=off  AntiWindupMode=back-calculation  Kb=1  TrackingMode=off  Kt=1  PParamMin=[]  PParamMax=[]  IParamMin=[]  IParamMax=[]  DParamMin=[]  DParamMax=[]  NParamMin=[]  NParamMax=[]  KbParamMin=[]  KbParamMax=[]  KtParamMin=[]  KtParamMax=[]  POutMin=[]  POutMax=[]  IOutMin=[]  IOutMax=[]  DOutMin=[]  DOutMax=[]  NOutMin=[]  NOutMax=[]  KbOutMin=[]  KbOutMax=[]  KtOutMin=[]  KtOutMax=[]  IntegratorOutMin=[]  IntegratorOutMax=[]  FilterOutMin=[]  FilterOutMax=[]  SumOutMin=[]  SumOutMax=[]  SumI1OutMin=[]  SumI1OutMax=[]  SumI2OutMin=[]  SumI2OutMax=[]  SumI3OutMin=[]  SumI3OutMax=[]  SumDOutMin=[]  SumDOutMax=[]  SaturationOutMin=[]  SaturationOutMax=[]  IntegratorContinuousStateAttributes=''  IntegratorStateMustResolveToSignalObject=off  IntegratorRTWStateStorageClass=Auto  FilterContinuousStateAttributes=''  FilterStateMustResolveToSignalObject=off  FilterRTWStateStorageClass=Auto
  Sum : Sum  Inputs=|-+
  Sum1 : Sum  Inputs=|-+
  w_ref (pu) : Outport
  V_ref (pu) : Outport  Port=2
  wires:
  Sum/1 -> Discrete PID Controller/1
  P (pu)/1 -> Sum/1
  Discrete PID Controller/1 -> w_ref (pu)/1
  P_ref (pu)/1 -> Sum/2
  Sum1/1 -> Discrete PID Controller1/1  "dq"
  Q (pu)/1 -> Sum1/1  "pu"
  Discrete PID Controller1/1 -> V_ref (pu)/1  "v"
  Q_ref (pu)/1 -> Sum1/2  "ref"

== system MODEL_FULL_SYSTEM/SM_Master/Generator_09222015/GenSet_4MVA_09212015/Simulated Generator Controller 3.5 MW/PV control ==
  P_ref (pu) : Inport
  P (pu) : Inport  Port=2
  Discrete PID Controller : simulink/Continuous/PID Controller  Controller=PID  TimeDomain=Discrete-time  SampleTime=-1  IntegratorMethod=Forward Euler  FilterMethod=Forward Euler  Form=Parallel  P=0.025  I=1  D=0  N=10  InitialConditionSource=internal  InitialConditionForIntegrator=0  InitialConditionForFilter=0  ExternalReset=none  LimitOutput=on  UpperSaturationLimit=1.15  LowerSaturationLimit=0.85  LinearizeAsGain=off  AntiWindupMode=back-calculation  Kb=1  TrackingMode=off  Kt=1  PParamMin=[]  PParamMax=[]  IParamMin=[]  IParamMax=[]  DParamMin=[]  DParamMax=[]  NParamMin=[]  NParamMax=[]  KbParamMin=[]  KbParamMax=[]  KtParamMin=[]  KtParamMax=[]  POutMin=[]  POutMax=[]  IOutMin=[]  IOutMax=[]  DOutMin=[]  DOutMax=[]  NOutMin=[]  NOutMax=[]  KbOutMin=[]  KbOutMax=[]  KtOutMin=[]  KtOutMax=[]  IntegratorOutMin=[]  IntegratorOutMax=[]  FilterOutMin=[]  FilterOutMax=[]  SumOutMin=[]  SumOutMax=[]  SumI1OutMin=[]  SumI1OutMax=[]  SumI2OutMin=[]  SumI2OutMax=[]  SumI3OutMin=[]  SumI3OutMax=[]  SumDOutMin=[]  SumDOutMax=[]  SaturationOutMin=[]  SaturationOutMax=[]  IntegratorContinuousStateAttributes=''  IntegratorStateMustResolveToSignalObject=off  IntegratorRTWStateStorageClass=Auto  FilterContinuousStateAttributes=''  FilterStateMustResolveToSignalObject=off  FilterRTWStateStorageClass=Auto
  Sum : Sum  Inputs=|-+
  w_ref (pu) : Outport
  wires:
  P_ref (pu)/1 -> Sum/2
  Discrete PID Controller/1 -> w_ref (pu)/1
  P (pu)/1 -> Sum/1
  Sum/1 -> Discrete PID Controller/1

== system MODEL_FULL_SYSTEM/SM_Master/Generator_09222015/Woodward Outputs/DIO - Gr3/Conditioning ==
  In1 : Inport
  Bus Creator : BusCreator  Inputs=8
  Demux : Demux  Outputs=8
  Out1 : Outport
  wires:
  Demux/1 -> Bus Creator/1  "Gen1_Starter"
  Demux/2 -> Bus Creator/2  "Gen1_Fuel"
  Demux/3 -> Bus Creator/3  "Gen1_Close_GCB"
  Demux/4 -> Bus Creator/4  "Gen1_Open_GCB"
  Demux/5 -> Bus Creator/5  "Gen1_Close_MCB"
  Demux/6 -> Bus Creator/6  "Gen1_Open_MCB"
  Demux/7 -> Bus Creator/7  "Gen1_Alarm_AB"
  Demux/8 -> Bus Creator/8  "Gen1_Alarm_CF"
  Bus Creator/1 -> Out1/1  "DI_CH00-07"
  In1/1 -> Demux/1

== system MODEL_FULL_SYSTEM/SM_Master/Generator_09222015/Woodward Outputs/DIO - Gr3/Conditioning1 ==
  In1 : Inport
  Bus Creator : BusCreator  Inputs=8
  Demux : Demux  Outputs=8
  Out1 : Outport
  wires:
  In1/1 -> Demux/1
  Bus Creator/1 -> Out1/1  "DI_CH08-15"
  Demux/8 -> Bus Creator/8  "Gen2_Alarm_CF"
  Demux/7 -> Bus Creator/7  "Gen2_Alarm_AB"
  Demux/6 -> Bus Creator/6  "Gen2_Open_MCB"
  Demux/5 -> Bus Creator/5  "Gen2_Close_MCB"
  Demux/4 -> Bus Creator/4  "Gen2_Open_GCB"
  Demux/3 -> Bus Creator/3  "Gen2_Close_GCB"
  Demux/2 -> Bus Creator/2  "Gen2_Fuel"
  Demux/1 -> Bus Creator/1  "Gen2_Starter"
